simulink model "Simulink_Part01"  (R2019a)
settings: Solver=VariableStepAuto  StartTime=0.0  StopTime=10.0  RelTol=1e-3
undefined symbols (not defined in the file): a1, a2
settings Model: Creator=Huyco  LastModifiedBy=Huyco

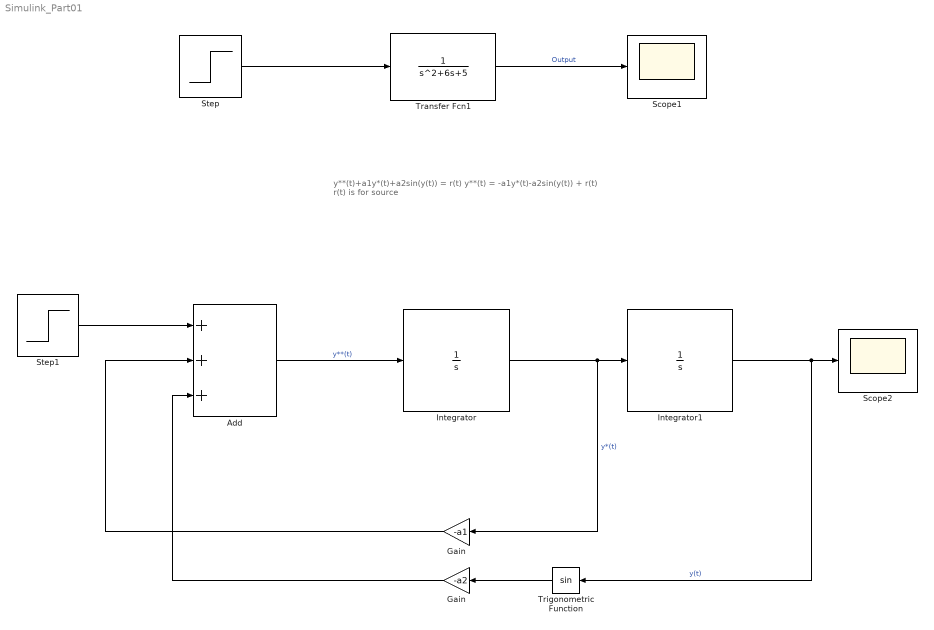
== system Simulink_Part01 ==
  note: y**(t)+a1y*(t)+a2sin(y(t)) = r(t)
      | y**(t) = -a1y*(t)-a2sin(y(t)) + r(t)
      | r(t) is for source
  Add : Sum  Inputs=3
  Gain : Gain  Gain=-a2
  "Gain " : Gain  Gain=-a1
  Integrator : Integrator
  Integrator1 : Integrator
  Scope1 : Scope
  Scope2 : Scope
  Step : Step  Time=0  SampleTime=0
  Step1 : Step  Time=0  SampleTime=0
  Transfer Fcn1 : TransferFcn  Denominator=[1 6 5]
  Trigonometric Function : Trigonometry
  wires:
  Step/1 -> Transfer Fcn1/1
  Transfer Fcn1/1 -> Scope1/1  "Output"
  Integrator/1 -> "Gain "/1, Integrator1/1  "y*(t)"
  Add/1 -> Integrator/1  "y**(t)"
  Integrator1/1 -> Trigonometric Function/1, Scope2/1  "y(t)"
  Gain/1 -> Add/3
  "Gain "/1 -> Add/2
  Trigonometric Function/1 -> Gain/1
  Step1/1 -> Add/1
